simulink model "Basic_cosimulation_circuit_simulator1"  (R2021b)
settings: Solver=ode4  StartTime=0.0  StopTime=inf  FixedStep=Ts  RelTol=1e-3  EnableMultiTasking=on
PostLoadFcn:
  | %
  | % Script for validation of swtiching model design with it's respective
  | % average model.
  | %
  | % Here it is presented the design of the inverter to the 6 kW Fuel Cell
  | % model.
  | 
  | %%% Initialization %%%
  | 
  | 
  | % ------------------------------------- %
  | % ---------- Inverter Design ---------- %
  | % ------------------------------------- %
  | 
  | %%%% Nominal Parameters %%%%
  | 
  | Pnom = 50e3;                                        % Nominal Power
  | Vdc = 400;                                          % DC Voltage - Boost
  | m = 0.6;                                            % Modulation Index
  | Vnom_peak = m*Vdc/2;                                % Peak Voltage
  | Vnom_rms = Vnom_peak/sqrt(2);                       % Rms Voltage
  | FP_min = 0.9;                                       % For Reactive Power
  |                                                     % Compensation
  | Snom = Pnom/FP_min;                                 % Apparent Power
  | Irms = Pnom/(sqrt(3)*Vnom_rms);                     % Rms Curren
  | Inom_peak = Irms*sqrt(2);                           % Peak Current
  | Zbase = Vnom_peak/Inom_peak;                        % Base Impedance
  | f = 60;                                             % Nominal Frequency
  | wnom = 2*pi*60;                                     % Angular Frequency
  | 
  | % ------------------------- %
  | % Inverter LC Filter Design %
  | % ------------------------- %
  | 
  | fsw_inv = 96*60;                                    % Switching Frequency must be a multiple of the nominal frequency
  |                                                      % for proper operation of the Artemis Block
  | ripple_inv = 0.03;
  | L_inv = ((Vdc/2)-Vnom_peak)*(1/fsw_inv)/(ripple_inv*Inom_peak);
  | 
  | % - Capacitor
  | fres = 420;                                         % Filters Ressonant Frequency
  | 
  | Cf = 1/(4*L_inv*(pi^2)*(fres^2));                % Filter Capacitor
  | Rf = 1/(wnom*Cf*50);                                % Damping Resistor
  | 
  | % --- Sample Time --- %
  | 
  | Tsw = 0.00050;
  | Ts = Tsw/10;
  | 
  | % ---------------------- %
  | % Current Control Design %
  | % ---------------------- %
  | 
  | Ron = 0.001;                                        % IGBT Resistance
  | tau_i = 1e-3;                                       % Responde Time
  | kp_current = L_inv/tau_i;                           % PI Proportional Gain
  | ki_current = (Ron)/tau_i;                           % PI Integral Gain
  | 
  | decouple = (wnom*L_inv);                            % Decoupling Gain
InitFcn:
  | %
  | % Script for validation of swtiching model design with it's respective
  | % average model.
  | %
  | % Here it is presented the design of the inverter to the 6 kW Fuel Cell
  | % model.
  | 
  | %%% Initialization %%%
  | 
  | 
  | % ------------------------------------- %
  | % ---------- Inverter Design ---------- %
  | % ------------------------------------- %
  | 
  | %%%% Nominal Parameters %%%%
  | 
  | Pnom = 50e3;                                        % Nominal Power
  | Vdc = 400;                                          % DC Voltage - Boost
  | m = 0.6;                                            % Modulation Index
  | Vnom_peak = m*Vdc/2;                                % Peak Voltage
  | Vnom_rms = Vnom_peak/sqrt(2);                       % Rms Voltage
  | FP_min = 0.9;                                       % For Reactive Power
  |                                                     % Compensation
  | Snom = Pnom/FP_min;                                 % Apparent Power
  | Irms = Pnom/(sqrt(3)*Vnom_rms);                     % Rms Curren
  | Inom_peak = Irms*sqrt(2);                           % Peak Current
  | Zbase = Vnom_peak/Inom_peak;                        % Base Impedance
  | f = 60;                                             % Nominal Frequency
  | wnom = 2*pi*60;                                     % Angular Frequency
  | 
  | % ------------------------- %
  | % Inverter LC Filter Design %
  | % ------------------------- %
  | 
  | fsw_inv = 96*60;                                    % Switching Frequency must be a multiple of the nominal frequency
  |                                                      % for proper operation of the Artemis Block
  | ripple_inv = 0.03;
  | L_inv = ((Vdc/2)-Vnom_peak)*(1/fsw_inv)/(ripple_inv*Inom_peak);
  | 
  | % - Capacitor
  | fres = 420;                                         % Filters Ressonant Frequency
  | 
  | Cf = 1/(4*L_inv*(pi^2)*(fres^2));                % Filter Capacitor
  | Rf = 1/(wnom*Cf*50);                                % Damping Resistor
  | 
  | % --- Sample Time --- %
  | 
  | Tsw = 0.00050;
  | Ts = Tsw/10;
  | 
  | % ---------------------- %
  | % Current Control Design %
  | % ---------------------- %
  | 
  | Ron = 0.001;                                        % IGBT Resistance
  | tau_i = 1e-3;                                       % Responde Time
  | kp_current = L_inv/tau_i;                           % PI Proportional Gain
  | ki_current = (Ron)/tau_i;                           % PI Integral Gain
  | 
  | decouple = (wnom*L_inv);                            % Decoupling Gain
undefined symbols (not defined in the file): D1, Delta, DiscIntNeverNeededParam, IP, j, ph, sps, UDP
libraries: spsCurrentMeasurementLib x25, spsControlledVoltageSourceLib x21, rtlab x18, spsGroundLib x13, spsThreePhaseSeriesRLCBranchLib x13, spsControlledCurrentSourceLib x11, spsVoltageMeasurementLib x10, simulink x8, rteventslib x8, powerlib_meascontrol x7, spsThreePhaseVIMeasurementLib x4, ssn_inverter_model x4
(part 4 of 5)

== system Basic_cosimulation_circuit_simulator1/SM_Master/Circuit_ITM_Source_DP_AW/DP - > EMT/Subsystem2 ==
  In1 : Inport
  Input2 : Inport  Port=2
  Compare To Constant : simulink/Logic and Bit Operations/Compare To Constant  relop=>=  const=2*pi  OutDataTypeStr=boolean
  Constant : Constant  Value=2*pi
  Constant2 : Constant  Value=2*pi*60
  Integrator : Integrator  ExternalReset=rising  InitialConditionSource=external  ShowStatePort=on
  Product4 : Product
  Sin3 : Trigonometry
  Sum : Sum  Inputs=|+-
  Sum4 : Sum  Inputs=|++
  Out1 : Outport
  wires:
  Product4/1 -> Out1/1
  In1/1 -> Product4/1
  Integrator/1 -> Sum4/2
  Input2/1 -> Sum4/1
  Sum4/1 -> Sin3/1
  Sin3/1 -> Product4/2
  Integrator/State -> Sum/1, Compare To Constant/1
  Constant2/1 -> Integrator/1
  Compare To Constant/1 -> Integrator/2
  Sum/1 -> Integrator/3
  Constant/1 -> Sum/2

== system Basic_cosimulation_circuit_simulator1/SM_Master/Original Circuit/Control/Current Control ==
  note: Block Inputs
  Deblock : Inport
  Idq_ref : Inport  Port=2
  Idq : Inport  Port=3
  Vdq : Inport  Port=4
  Phase : Inport  Port=5
  Constant2 : Constant  Value=Vdc/2
  Delay : Delay  DelayLength=1
  Demux1 : Demux  Outputs=2
  Demux2 : Demux  Outputs=2
  Demux3 : Demux  Outputs=2
  Discrete-Time Integrator : DiscreteIntegrator  SampleTime=-1  ICPrevOutput=DiscIntNeverNeededParam  ICPrevScaledInput=DiscIntNeverNeededParam
  Discrete-Time Integrator1 : DiscreteIntegrator  SampleTime=-1  ICPrevOutput=DiscIntNeverNeededParam  ICPrevScaledInput=DiscIntNeverNeededParam
  Divide : Product  Inputs=*/
  Divide1 : Product  Inputs=*/
  Gain1 : Gain  Gain=kp_current
  Gain2 : Gain  Gain=ki_current
  Gain3 : Gain  Gain=kp_current
  Gain4 : Gain  Gain=ki_current
  Gain5 : Gain  Gain=decouple
  Gain6 : Gain  Gain=decouple
  Inverse_Park_Transformation : Subsystem
  Mux : Mux  Inputs=2
  Product : Product
  Product1 : Product
  Saturation : Saturate  UpperLimit=1.2*Inom_peak  LowerLimit=-1.2*Inom_peak
  Saturation1 : Saturate  UpperLimit=1.2*Inom_peak  LowerLimit=-1.2*Inom_peak
  Subtract : Sum  Inputs=+-
  Subtract1 : Sum  Inputs=+-
  Sum1 : Sum
  Sum2 : Sum
  Sum3 : Sum  Inputs=++-
  Sum4 : Sum  Inputs=+++
  modulation : Outport
  wires:
  Sum4/1 -> Divide1/1
  Sum3/1 -> Divide/1
  Sum2/1 -> Sum4/2
  Subtract/1 -> Product/1
  Gain2/1 -> Discrete-Time Integrator/1
  [Iq] -> Gain5/1
  Gain1/1 -> Sum1/1
  [Id] -> Gain6/1
  Subtract1/1 -> Product1/2
  Gain6/1 -> Sum4/1
  Product/1 -> Gain2/1, Gain1/1
  [Vd] -> Sum3/1
  Constant2/1 -> Divide1/2, Divide/2
  Idq_ref/1 -> Demux3/1
  Mux/1 -> Delay/1
  Gain5/1 -> Sum3/3
  Sum1/1 -> Sum3/2
  Discrete-Time Integrator/1 -> Sum1/2
  Gain3/1 -> Sum2/1
  Gain4/1 -> Discrete-Time Integrator1/1
  Discrete-Time Integrator1/1 -> Sum2/2
  [Vq] -> Sum4/3
  Product1/1 -> Gain3/1, Gain4/1
  [Id] -> Subtract/2
  Divide/1 -> Mux/1
  Divide1/1 -> Mux/2
  [Iq] -> Subtract1/2
  Inverse_Park_Transformation/1(ABC) -> modulation/1
  Idq/1 -> Demux1/1
  Demux1/1 -> [Id]
  Demux1/2 -> [Iq]
  Demux2/1 -> [Vd]
  Demux2/2 -> [Vq]
  Vdq/1 -> Demux2/1
  [dblk] -> Product1/1, Product/2
  Deblock/1 -> [dblk]
  Phase/1 -> [phase_pll]
  [phase_pll] -> Inverse_Park_Transformation/2(Phase)
  Demux3/1 -> [Id_ref]
  Demux3/2 -> [Iq_ref]
  [Iq_ref] -> Saturation1/1
  [Id_ref] -> Saturation/1
  Saturation/1 -> Subtract/1
  Saturation1/1 -> Subtract1/1
  Delay/1 -> Inverse_Park_Transformation/1(DQ)

== system Basic_cosimulation_circuit_simulator1/SM_Master/Original Circuit/Control/Meas_3_Wire ==
  AB : Inport
  BC : Inport  Port=2
  Gain10 : Gain  Gain=2
  Gain6 : Gain  Gain=2
  Gain7 : Gain  Gain=1/3
  Gain8 : Gain  Gain=1/3
  Gain9 : Gain  Gain=1/3
  Mux : Mux  Inputs=3
  Sum4 : Sum  Inputs=|++
  Sum5 : Sum  Inputs=-+|
  Sum6 : Sum  Inputs=--|
  ABC : Outport
  wires:
  BC/1 -> Sum4/2, Sum5/2, Gain10/1
  AB/1 -> Gain6/1, Sum5/1, Sum6/2
  Gain7/1 -> Mux/1
  Gain9/1 -> Mux/3
  Sum6/1 -> Gain9/1
  Gain6/1 -> Sum4/1
  Gain8/1 -> Mux/2
  Sum5/1 -> Gain8/1
  Gain10/1 -> Sum6/1
  Sum4/1 -> Gain7/1
  Mux/1 -> ABC/1

== system Basic_cosimulation_circuit_simulator1/SM_Master/Original Circuit/Control/Park_Transformation ==
  note: Park Transformation
  ABC : Inport
  Phase : Inport  Port=2
  Constant{,1..3} (4 alike) : Constant  Value=2*pi/3
  Cos : Trigonometry  Operator=cos
  Cos1 : Trigonometry  Operator=cos
  Cos2 : Trigonometry  Operator=cos
  Cos3 : Trigonometry
  Cos4 : Trigonometry
  Cos5 : Trigonometry
  Delay : Delay  DelayLength=1
  Demux : Demux  Outputs=3
  Gain : Gain  Gain=0.666
  Gain1 : Gain  Gain=-0.666
  Mux : Mux  Inputs=2
  Product{,1..5} (6 alike) : Product
  Sum : Sum  Inputs=|+-
  Sum1 : Sum  Inputs=+++
  Sum2 : Sum  Inputs=|++
  Sum3 : Sum  Inputs=|+-
  Sum4 : Sum  Inputs=+++
  Sum5 : Sum  Inputs=|++
  DQ : Outport
  wires:
  ABC/1 -> Demux/1
  Demux/1 -> [A]
  Demux/2 -> [B]
  Demux/3 -> [C]
  Phase/1 -> [phase]
  [A] -> Product/1
  [phase] -> Cos/1
  Cos/1 -> Product/2
  Product/1 -> Sum1/1
  [B] -> Product1/1
  Product1/1 -> Sum1/2
  [phase] -> Sum/1
  Constant/1 -> Sum/2
  Sum/1 -> Cos1/1
  Cos1/1 -> Product1/2
  Sum2/1 -> Cos2/1
  Constant1/1 -> Sum2/2
  Cos2/1 -> Product2/2
  [phase] -> Sum2/1
  [C] -> Product2/1
  Product2/1 -> Sum1/3
  Sum4/1 -> Gain1/1
  Product5/1 -> Sum4/3
  [C] -> Product5/1
  [phase] -> Sum5/1
  Cos5/1 -> Product5/2
  Constant3/1 -> Sum5/2
  Sum5/1 -> Cos5/1
  Cos4/1 -> Product4/2
  Sum3/1 -> Cos4/1
  Constant2/1 -> Sum3/2
  [phase] -> Sum3/1
  Product4/1 -> Sum4/2
  [B] -> Product4/1
  Product3/1 -> Sum4/1
  Cos3/1 -> Product3/2
  [phase] -> Cos3/1
  [A] -> Product3/1
  Sum1/1 -> Gain/1
  Gain/1 -> [D]
  Gain1/1 -> [Q]
  [D] -> Mux/1
  [Q] -> Mux/2
  Mux/1 -> Delay/1
  Delay/1 -> DQ/1

== system Basic_cosimulation_circuit_simulator1/SM_Master/Original Circuit/Control/Park_Transformation1 ==
  note: Park Transformation
  ABC : Inport
  Phase : Inport  Port=2
  Constant{,1..3} (4 alike) : Constant  Value=2*pi/3
  Cos : Trigonometry  Operator=cos
  Cos1 : Trigonometry  Operator=cos
  Cos2 : Trigonometry  Operator=cos
  Cos3 : Trigonometry
  Cos4 : Trigonometry
  Cos5 : Trigonometry
  Delay : Delay  DelayLength=1
  Demux : Demux  Outputs=3
  Gain : Gain  Gain=0.666
  Gain1 : Gain  Gain=-0.666
  Mux : Mux  Inputs=2
  Product{,1..5} (6 alike) : Product
  Sum : Sum  Inputs=|+-
  Sum1 : Sum  Inputs=+++
  Sum2 : Sum  Inputs=|++
  Sum3 : Sum  Inputs=|+-
  Sum4 : Sum  Inputs=+++
  Sum5 : Sum  Inputs=|++
  DQ : Outport
  wires:
  [Q] -> Mux/2
  [D] -> Mux/1
  Gain1/1 -> [Q]
  Gain/1 -> [D]
  Sum1/1 -> Gain/1
  [A] -> Product3/1
  [phase] -> Cos3/1
  Cos3/1 -> Product3/2
  Product3/1 -> Sum4/1
  [B] -> Product4/1
  Product4/1 -> Sum4/2
  [phase] -> Sum3/1
  Constant2/1 -> Sum3/2
  Sum3/1 -> Cos4/1
  Cos4/1 -> Product4/2
  Sum5/1 -> Cos5/1
  Constant3/1 -> Sum5/2
  Cos5/1 -> Product5/2
  [phase] -> Sum5/1
  [C] -> Product5/1
  Product5/1 -> Sum4/3
  Sum4/1 -> Gain1/1
  Product2/1 -> Sum1/3
  [C] -> Product2/1
  [phase] -> Sum2/1
  Cos2/1 -> Product2/2
  Constant1/1 -> Sum2/2
  Sum2/1 -> Cos2/1
  Cos1/1 -> Product1/2
  Sum/1 -> Cos1/1
  Constant/1 -> Sum/2
  [phase] -> Sum/1
  Product1/1 -> Sum1/2
  [B] -> Product1/1
  Product/1 -> Sum1/1
  Cos/1 -> Product/2
  [phase] -> Cos/1
  [A] -> Product/1
  Phase/1 -> [phase]
  Demux/3 -> [C]
  Demux/2 -> [B]
  Demux/1 -> [A]
  ABC/1 -> Demux/1
  Mux/1 -> Delay/1
  Delay/1 -> DQ/1

== system Basic_cosimulation_circuit_simulator1/SM_Master/Original Circuit/Control/Power Control ==
  PQ_ref : Inport
  Vd : Inport  Port=2
  Dblk : Inport  Port=3
  Constant : Constant  Value=Vnom_peak
  Demux2 : Demux  Outputs=2
  Divide : Product  Inputs=*/
  Divide1 : Product  Inputs=*/
  Gain : Gain  Gain=3
  Gain1 : Gain  Gain=2
  Gain2 : Gain  Gain=3
  Gain3 : Gain  Gain=-2
  Mux : Mux  Inputs=2
  Scope : Scope
  Switch : Switch  Criteria=u2 > Threshold
  Transfer Fcn : TransferFcn  Commented=on  Denominator=[0.01 1]
  Out1 : Outport
  wires:
  Gain/1 -> Divide/2
  Demux2/2 -> Gain3/1
  Gain2/1 -> Divide1/2
  Gain3/1 -> Divide1/1
  Demux2/1 -> Gain1/1
  Dblk/1 -> Switch/2
  Gain1/1 -> Divide/1
  Divide/1 -> Mux/1
  Constant/1 -> Switch/3
  [Vd_power] -> Gain/1
  Divide1/1 -> Mux/2
  Mux/1 -> Out1/1
  PQ_ref/1 -> Demux2/1
  Vd/1 -> Switch/1
  Switch/1 -> Scope/1, Gain2/1, [Vd_power]

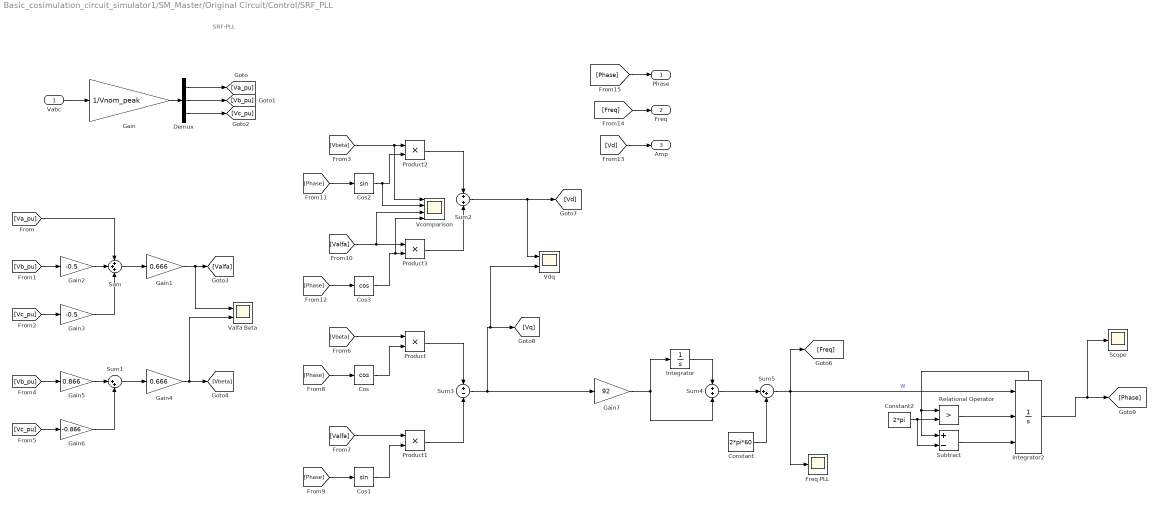
== system Basic_cosimulation_circuit_simulator1/SM_Master/Original Circuit/Control/SRF_PLL ==
  note: SRF-PLL
  Vabc : Inport
  Constant : Constant  Value=2*pi*60
  Constant2 : Constant  Value=2*pi
  Cos : Trigonometry  Operator=cos
  Cos1 : Trigonometry
  Cos2 : Trigonometry
  Cos3 : Trigonometry  Operator=cos
  Demux : Demux  Outputs=3
  Freq PLL : Scope
  Gain : Gain  Gain=1/Vnom_peak
  Gain1 : Gain  Gain=0.666
  Gain2 : Gain  Gain=-0.5
  Gain3 : Gain  Gain=-0.5
  Gain4 : Gain  Gain=0.666
  Gain5 : Gain  Gain=0.866
  Gain6 : Gain  Gain=-0.866
  Gain7 : Gain  Gain=92
  Integrator : Integrator
  Integrator2 : Integrator  ExternalReset=rising  InitialConditionSource=external  InitialCondition=sps.Phase_Init*pi/180  LimitOutput=on  ShowStatePort=on
  Product{,1..3} (4 alike) : Product
  Relational Operator : RelationalOperator  Operator=>  OutDataTypeStr=boolean  RndMeth=Nearest
  Scope : Scope
  Subtract : Sum  Inputs=+-
  Sum : Sum  Inputs=+++
  Sum1 : Sum  Inputs=|++
  Sum2 : Sum  Inputs=+|+
  Sum3 : Sum  Inputs=+|-
  Sum4 : Sum  Inputs=+|+
  Sum5 : Sum  Inputs=|++
  Valfa Beta : Scope  NumInputPorts=2
  Vcomparison : Scope  NumInputPorts=4
  Vdq : Scope  NumInputPorts=2
  Phase : Outport
  Freq : Outport  Port=2
  Amp : Outport  Port=3
  wires:
  Vabc/1 -> Gain/1
  Demux/1 -> [Va_pu]
  Demux/2 -> [Vb_pu]
  Demux/3 -> [Vc_pu]
  Gain/1 -> Demux/1
  Sum/1 -> Gain1/1
  [Va_pu] -> Sum/1
  [Vb_pu] -> Gain2/1
  Gain2/1 -> Sum/2
  [Vc_pu] -> Gain3/1
  Gain3/1 -> Sum/3
  [Vc_pu] -> Gain6/1
  [Vb_pu] -> Gain5/1
  Sum1/1 -> Gain4/1
  Gain4/1 -> Valfa Beta/2, [Vbeta]
  Gain5/1 -> Sum1/1
  Gain6/1 -> Sum1/2
  [Vbeta] -> Product/1
  Product/1 -> Sum3/1
  [Valfa] -> Product1/1
  Product1/1 -> Sum3/2
  Sum3/1 -> Gain7/1, Vdq/2, [Vq]
  Gain7/1 -> Sum4/2, Integrator/1
  Integrator/1 -> Sum4/1
  Sum4/1 -> Sum5/1
  Constant/1 -> Sum5/2
  [Phase] -> Cos/1
  Cos/1 -> Product/2
  [Phase] -> Cos1/1
  Cos1/1 -> Product1/2
  Cos3/1 -> Vcomparison/4, Product3/2
  [Phase] -> Cos3/1
  Cos2/1 -> Vcomparison/2, Product2/2
  [Phase] -> Cos2/1
  Product3/1 -> Sum2/2
  [Valfa] -> Vcomparison/3, Product3/1
  Product2/1 -> Sum2/1
  [Vbeta] -> Vcomparison/1, Product2/1
  [Vd] -> Amp/1
  [Freq] -> Freq/1
  [Phase] -> Phase/1
  Gain1/1 -> Valfa Beta/1, [Valfa]
  Sum2/1 -> Vdq/1, [Vd]
  Integrator2/1 -> Scope/1, [Phase]
  Subtract/1 -> Integrator2/3
  Integrator2/State -> Relational Operator/1, Subtract/1
  Sum5/1 -> Integrator2/1, Freq PLL/1, [Freq]  "W"
  Relational Operator/1 -> Integrator2/2
  Constant2/1 -> Relational Operator/2, Subtract/2

== system Basic_cosimulation_circuit_simulator1/SM_Master/VSC_ITM_Average_Moving_Window/Control/Current Control ==
  note: Block Inputs
  Deblock : Inport
  Idq_ref : Inport  Port=2
  Idq : Inport  Port=3
  Vdq : Inport  Port=4
  Phase : Inport  Port=5
  Constant2 : Constant  Value=Vdc/2
  Delay : Delay  DelayLength=1
  Demux1 : Demux  Outputs=2
  Demux2 : Demux  Outputs=2
  Demux3 : Demux  Outputs=2
  Discrete-Time Integrator : DiscreteIntegrator  SampleTime=-1  ICPrevOutput=DiscIntNeverNeededParam  ICPrevScaledInput=DiscIntNeverNeededParam
  Discrete-Time Integrator1 : DiscreteIntegrator  SampleTime=-1  ICPrevOutput=DiscIntNeverNeededParam  ICPrevScaledInput=DiscIntNeverNeededParam
  Divide : Product  Inputs=*/
  Divide1 : Product  Inputs=*/
  Gain1 : Gain  Gain=kp_current
  Gain2 : Gain  Gain=ki_current
  Gain3 : Gain  Gain=kp_current
  Gain4 : Gain  Gain=ki_current
  Gain5 : Gain  Gain=decouple
  Gain6 : Gain  Gain=decouple
  Inverse_Park_Transformation : Subsystem
  Mux : Mux  Inputs=2
  Product : Product
  Product1 : Product
  Saturation : Saturate  UpperLimit=1.2*Inom_peak  LowerLimit=-1.2*Inom_peak
  Saturation1 : Saturate  UpperLimit=1.2*Inom_peak  LowerLimit=-1.2*Inom_peak
  Scope : Scope  Commented=on
  Subtract : Sum  Inputs=+-
  Subtract1 : Sum  Inputs=+-
  Sum1 : Sum
  Sum2 : Sum
  Sum3 : Sum  Inputs=++-
  Sum4 : Sum  Inputs=+++
  modulation : Outport
  wires:
  Sum4/1 -> Divide1/1
  Sum3/1 -> Divide/1
  Sum2/1 -> Sum4/2
  Subtract/1 -> Product/1
  Gain2/1 -> Discrete-Time Integrator/1
  [Iq] -> Gain5/1
  Gain1/1 -> Sum1/1
  [Id] -> Gain6/1
  Subtract1/1 -> Product1/2
  Gain6/1 -> Sum4/1
  Product/1 -> Gain2/1, Gain1/1
  [Vd] -> Sum3/1
  Constant2/1 -> Divide1/2, Divide/2
  Idq_ref/1 -> Demux3/1
  Mux/1 -> Delay/1
  Gain5/1 -> Sum3/3
  Sum1/1 -> Sum3/2
  Discrete-Time Integrator/1 -> Sum1/2
  Gain3/1 -> Sum2/1
  Gain4/1 -> Discrete-Time Integrator1/1
  Discrete-Time Integrator1/1 -> Sum2/2
  [Vq] -> Sum4/3
  Product1/1 -> Gain3/1, Gain4/1
  [Id] -> Subtract/2
  Divide/1 -> Mux/1
  Divide1/1 -> Mux/2
  [Iq] -> Subtract1/2
  Inverse_Park_Transformation/1(ABC) -> modulation/1
  Idq/1 -> Demux1/1
  Demux1/1 -> [Id]
  Demux1/2 -> [Iq]
  Demux2/1 -> [Vd]
  Demux2/2 -> [Vq]
  Vdq/1 -> Demux2/1
  [dblk] -> Product1/1, Product/2
  Deblock/1 -> [dblk]
  Phase/1 -> [phase_pll]
  [phase_pll] -> Inverse_Park_Transformation/2(Phase)
  Demux3/1 -> [Id_ref]
  Demux3/2 -> [Iq_ref]
  [Iq_ref] -> Saturation1/1
  [Id_ref] -> Saturation/1
  Saturation/1 -> Subtract/1
  Saturation1/1 -> Subtract1/1
  Delay/1 -> Scope/1, Inverse_Park_Transformation/1(DQ)

== system Basic_cosimulation_circuit_simulator1/SM_Master/VSC_ITM_Average_Moving_Window/Control/Meas_3_Wire ==
  AB : Inport
  BC : Inport  Port=2
  Gain10 : Gain  Gain=2
  Gain6 : Gain  Gain=2
  Gain7 : Gain  Gain=1/3
  Gain8 : Gain  Gain=1/3
  Gain9 : Gain  Gain=1/3
  Mux : Mux  Inputs=3
  Sum4 : Sum  Inputs=|++
  Sum5 : Sum  Inputs=-+|
  Sum6 : Sum  Inputs=--|
  ABC : Outport
  wires:
  BC/1 -> Sum4/2, Sum5/2, Gain10/1
  AB/1 -> Gain6/1, Sum5/1, Sum6/2
  Gain7/1 -> Mux/1
  Gain9/1 -> Mux/3
  Sum6/1 -> Gain9/1
  Gain6/1 -> Sum4/1
  Gain8/1 -> Mux/2
  Sum5/1 -> Gain8/1
  Gain10/1 -> Sum6/1
  Sum4/1 -> Gain7/1
  Mux/1 -> ABC/1

== system Basic_cosimulation_circuit_simulator1/SM_Master/VSC_ITM_Average_Moving_Window/Control/Park_Transformation ==
  note: Park Transformation
  ABC : Inport
  Phase : Inport  Port=2
  Constant{,1..3} (4 alike) : Constant  Value=2*pi/3
  Cos : Trigonometry  Operator=cos
  Cos1 : Trigonometry  Operator=cos
  Cos2 : Trigonometry  Operator=cos
  Cos3 : Trigonometry
  Cos4 : Trigonometry
  Cos5 : Trigonometry
  Delay : Delay  DelayLength=1
  Demux : Demux  Outputs=3
  Gain : Gain  Gain=0.666
  Gain1 : Gain  Gain=-0.666
  Mux : Mux  Inputs=2
  Product{,1..5} (6 alike) : Product
  Sum : Sum  Inputs=|+-
  Sum1 : Sum  Inputs=+++
  Sum2 : Sum  Inputs=|++
  Sum3 : Sum  Inputs=|+-
  Sum4 : Sum  Inputs=+++
  Sum5 : Sum  Inputs=|++
  DQ : Outport
  wires:
  ABC/1 -> Demux/1
  Demux/1 -> [A]
  Demux/2 -> [B]
  Demux/3 -> [C]
  Phase/1 -> [phase]
  [A] -> Product/1
  [phase] -> Cos/1
  Cos/1 -> Product/2
  Product/1 -> Sum1/1
  [B] -> Product1/1
  Product1/1 -> Sum1/2
  [phase] -> Sum/1
  Constant/1 -> Sum/2
  Sum/1 -> Cos1/1
  Cos1/1 -> Product1/2
  Sum2/1 -> Cos2/1
  Constant1/1 -> Sum2/2
  Cos2/1 -> Product2/2
  [phase] -> Sum2/1
  [C] -> Product2/1
  Product2/1 -> Sum1/3
  Sum4/1 -> Gain1/1
  Product5/1 -> Sum4/3
  [C] -> Product5/1
  [phase] -> Sum5/1
  Cos5/1 -> Product5/2
  Constant3/1 -> Sum5/2
  Sum5/1 -> Cos5/1
  Cos4/1 -> Product4/2
  Sum3/1 -> Cos4/1
  Constant2/1 -> Sum3/2
  [phase] -> Sum3/1
  Product4/1 -> Sum4/2
  [B] -> Product4/1
  Product3/1 -> Sum4/1
  Cos3/1 -> Product3/2
  [phase] -> Cos3/1
  [A] -> Product3/1
  Sum1/1 -> Gain/1
  Gain/1 -> [D]
  Gain1/1 -> [Q]
  [D] -> Mux/1
  [Q] -> Mux/2
  Mux/1 -> Delay/1
  Delay/1 -> DQ/1

== system Basic_cosimulation_circuit_simulator1/SM_Master/VSC_ITM_Average_Moving_Window/Control/Park_Transformation1 ==
  note: Park Transformation
  ABC : Inport
  Phase : Inport  Port=2
  Constant{,1..3} (4 alike) : Constant  Value=2*pi/3
  Cos : Trigonometry  Operator=cos
  Cos1 : Trigonometry  Operator=cos
  Cos2 : Trigonometry  Operator=cos
  Cos3 : Trigonometry
  Cos4 : Trigonometry
  Cos5 : Trigonometry
  Delay : Delay  DelayLength=1
  Demux : Demux  Outputs=3
  Gain : Gain  Gain=0.666
  Gain1 : Gain  Gain=-0.666
  Mux : Mux  Inputs=2
  Product{,1..5} (6 alike) : Product
  Sum : Sum  Inputs=|+-
  Sum1 : Sum  Inputs=+++
  Sum2 : Sum  Inputs=|++
  Sum3 : Sum  Inputs=|+-
  Sum4 : Sum  Inputs=+++
  Sum5 : Sum  Inputs=|++
  DQ : Outport
  wires:
  [Q] -> Mux/2
  [D] -> Mux/1
  Gain1/1 -> [Q]
  Gain/1 -> [D]
  Sum1/1 -> Gain/1
  [A] -> Product3/1
  [phase] -> Cos3/1
  Cos3/1 -> Product3/2
  Product3/1 -> Sum4/1
  [B] -> Product4/1
  Product4/1 -> Sum4/2
  [phase] -> Sum3/1
  Constant2/1 -> Sum3/2
  Sum3/1 -> Cos4/1
  Cos4/1 -> Product4/2
  Sum5/1 -> Cos5/1
  Constant3/1 -> Sum5/2
  Cos5/1 -> Product5/2
  [phase] -> Sum5/1
  [C] -> Product5/1
  Product5/1 -> Sum4/3
  Sum4/1 -> Gain1/1
  Product2/1 -> Sum1/3
  [C] -> Product2/1
  [phase] -> Sum2/1
  Cos2/1 -> Product2/2
  Constant1/1 -> Sum2/2
  Sum2/1 -> Cos2/1
  Cos1/1 -> Product1/2
  Sum/1 -> Cos1/1
  Constant/1 -> Sum/2
  [phase] -> Sum/1
  Product1/1 -> Sum1/2
  [B] -> Product1/1
  Product/1 -> Sum1/1
  Cos/1 -> Product/2
  [phase] -> Cos/1
  [A] -> Product/1
  Phase/1 -> [phase]
  Demux/3 -> [C]
  Demux/2 -> [B]
  Demux/1 -> [A]
  ABC/1 -> Demux/1
  Mux/1 -> Delay/1
  Delay/1 -> DQ/1

== system Basic_cosimulation_circuit_simulator1/SM_Master/VSC_ITM_Average_Moving_Window/Control/Power Control ==
  PQ_ref : Inport
  Vd : Inport  Port=2
  Dblk : Inport  Port=3
  Constant : Constant  Value=Vnom_peak
  Demux2 : Demux  Outputs=2
  Divide : Product  Inputs=*/
  Divide1 : Product  Inputs=*/
  Gain : Gain  Gain=3
  Gain1 : Gain  Gain=2
  Gain2 : Gain  Gain=3
  Gain3 : Gain  Gain=-2
  Mux : Mux  Inputs=2
  Scope : Scope
  Switch : Switch  Criteria=u2 > Threshold
  Transfer Fcn : TransferFcn  Commented=on  Denominator=[0.01 1]
  Out1 : Outport
  wires:
  Gain/1 -> Divide/2
  Demux2/2 -> Gain3/1
  Gain2/1 -> Divide1/2
  Gain3/1 -> Divide1/1
  Demux2/1 -> Gain1/1
  Dblk/1 -> Switch/2
  Gain1/1 -> Divide/1
  Divide/1 -> Mux/1
  Constant/1 -> Switch/3
  [Vd_power] -> Gain/1
  Divide1/1 -> Mux/2
  Mux/1 -> Out1/1
  PQ_ref/1 -> Demux2/1
  Vd/1 -> Switch/1
  Switch/1 -> Scope/1, Gain2/1, [Vd_power]

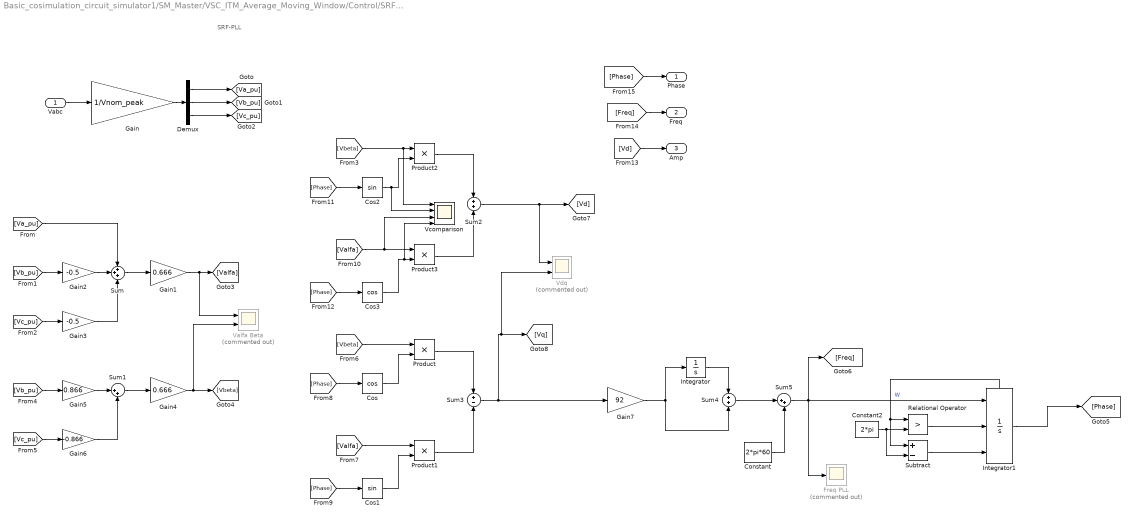
== system Basic_cosimulation_circuit_simulator1/SM_Master/VSC_ITM_Average_Moving_Window/Control/SRF_PLL ==
  note: SRF-PLL
  Vabc : Inport
  Constant : Constant  Value=2*pi*60
  Constant2 : Constant  Value=2*pi
  Cos : Trigonometry  Operator=cos
  Cos1 : Trigonometry
  Cos2 : Trigonometry
  Cos3 : Trigonometry  Operator=cos
  Demux : Demux  Outputs=3
  Freq PLL : Scope  Commented=on
  Gain : Gain  Gain=1/Vnom_peak
  Gain1 : Gain  Gain=0.666
  Gain2 : Gain  Gain=-0.5
  Gain3 : Gain  Gain=-0.5
  Gain4 : Gain  Gain=0.666
  Gain5 : Gain  Gain=0.866
  Gain6 : Gain  Gain=-0.866
  Gain7 : Gain  Gain=92
  Integrator : Integrator
  Integrator1 : Integrator  ExternalReset=rising  InitialConditionSource=external  InitialCondition=sps.Phase_Init*pi/180  LimitOutput=on  ShowStatePort=on
  Product{,1..3} (4 alike) : Product
  Relational Operator : RelationalOperator  Operator=>  OutDataTypeStr=boolean  RndMeth=Nearest
  Subtract : Sum  Inputs=+-
  Sum : Sum  Inputs=+++
  Sum1 : Sum  Inputs=|++
  Sum2 : Sum  Inputs=+|+
  Sum3 : Sum  Inputs=+|-
  Sum4 : Sum  Inputs=+|+
  Sum5 : Sum  Inputs=|++
  Valfa Beta : Scope  Commented=on  NumInputPorts=2
  Vcomparison : Scope  NumInputPorts=4
  Vdq : Scope  Commented=on  NumInputPorts=2
  Phase : Outport
  Freq : Outport  Port=2
  Amp : Outport  Port=3
  wires:
  Vabc/1 -> Gain/1
  Demux/1 -> [Va_pu]
  Demux/2 -> [Vb_pu]
  Demux/3 -> [Vc_pu]
  Gain/1 -> Demux/1
  Sum/1 -> Gain1/1
  [Va_pu] -> Sum/1
  [Vb_pu] -> Gain2/1
  Gain2/1 -> Sum/2
  [Vc_pu] -> Gain3/1
  Gain3/1 -> Sum/3
  [Vc_pu] -> Gain6/1
  [Vb_pu] -> Gain5/1
  Sum1/1 -> Gain4/1
  Gain4/1 -> Valfa Beta/2, [Vbeta]
  Gain5/1 -> Sum1/1
  Gain6/1 -> Sum1/2
  [Vbeta] -> Product/1
  Product/1 -> Sum3/1
  [Valfa] -> Product1/1
  Product1/1 -> Sum3/2
  Sum3/1 -> Gain7/1, Vdq/2, [Vq]
  Gain7/1 -> Sum4/2, Integrator/1
  Integrator/1 -> Sum4/1
  Sum4/1 -> Sum5/1
  Constant/1 -> Sum5/2
  [Phase] -> Cos/1
  Cos/1 -> Product/2
  [Phase] -> Cos1/1
  Cos1/1 -> Product1/2
  Cos3/1 -> Vcomparison/4, Product3/2
  [Phase] -> Cos3/1
  Cos2/1 -> Vcomparison/2, Product2/2
  [Phase] -> Cos2/1
  Product3/1 -> Sum2/2
  [Valfa] -> Vcomparison/3, Product3/1
  Product2/1 -> Sum2/1
  [Vbeta] -> Vcomparison/1, Product2/1
  [Vd] -> Amp/1
  [Freq] -> Freq/1
  [Phase] -> Phase/1
  Gain1/1 -> Valfa Beta/1, [Valfa]
  Sum2/1 -> Vdq/1, [Vd]
  Constant2/1 -> Relational Operator/2, Subtract/2
  Integrator1/State -> Relational Operator/1, Subtract/1
  Sum5/1 -> Integrator1/1, Freq PLL/1, [Freq]  "W"
  Relational Operator/1 -> Integrator1/2
  Subtract/1 -> Integrator1/3
  Integrator1/1 -> [Phase]

== system Basic_cosimulation_circuit_simulator1/SM_Master/VSC_ITM_Average_Moving_Window/DP - > EMT/Subsystem ==
  In1 : Inport
  Input : Inport  Port=2
  Compare To Constant : simulink/Logic and Bit Operations/Compare To Constant  relop=>=  const=2*pi  OutDataTypeStr=boolean
  Constant : Constant  Value=2*pi
  Constant2 : Constant  Value=2*pi*60
  Integrator : Integrator  ExternalReset=rising  InitialConditionSource=external  ShowStatePort=on
  Product4 : Product
  Sin3 : Trigonometry
  Sum : Sum  Inputs=|+-
  Sum4 : Sum  Inputs=|++
  Out1 : Outport
  wires:
  Product4/1 -> Out1/1
  In1/1 -> Product4/1
  Integrator/1 -> Sum4/2
  Input/1 -> Sum4/1
  Sum4/1 -> Sin3/1
  Sin3/1 -> Product4/2
  Integrator/State -> Sum/1, Compare To Constant/1
  Constant2/1 -> Integrator/1
  Compare To Constant/1 -> Integrator/2
  Sum/1 -> Integrator/3
  Constant/1 -> Sum/2

== system Basic_cosimulation_circuit_simulator1/SM_Master/VSC_ITM_Average_Moving_Window/DP - > EMT/Subsystem1 ==
  In1 : Inport
  Input1 : Inport  Port=2
  Compare To Constant : simulink/Logic and Bit Operations/Compare To Constant  relop=>=  const=2*pi  OutDataTypeStr=boolean
  Constant : Constant  Value=2*pi
  Constant2 : Constant  Value=2*pi*60
  Integrator : Integrator  ExternalReset=rising  InitialConditionSource=external  ShowStatePort=on
  Product4 : Product
  Sin3 : Trigonometry
  Sum : Sum  Inputs=|+-
  Sum4 : Sum  Inputs=|++
  Out1 : Outport
  wires:
  Product4/1 -> Out1/1
  In1/1 -> Product4/1
  Integrator/1 -> Sum4/2
  Input1/1 -> Sum4/1
  Sum4/1 -> Sin3/1
  Sin3/1 -> Product4/2
  Constant/1 -> Sum/2
  Sum/1 -> Integrator/3
  Compare To Constant/1 -> Integrator/2
  Integrator/State -> Sum/1, Compare To Constant/1
  Constant2/1 -> Integrator/1

== system Basic_cosimulation_circuit_simulator1/SM_Master/VSC_ITM_Average_Moving_Window/DP - > EMT/Subsystem2 ==
  In1 : Inport
  Input2 : Inport  Port=2
  Compare To Constant : simulink/Logic and Bit Operations/Compare To Constant  relop=>=  const=2*pi  OutDataTypeStr=boolean
  Constant : Constant  Value=2*pi
  Constant2 : Constant  Value=2*pi*60
  Integrator : Integrator  ExternalReset=rising  InitialConditionSource=external  ShowStatePort=on
  Product4 : Product
  Sin3 : Trigonometry
  Sum : Sum  Inputs=|+-
  Sum4 : Sum  Inputs=|++
  Out1 : Outport
  wires:
  Product4/1 -> Out1/1
  In1/1 -> Product4/1
  Integrator/1 -> Sum4/2
  Input2/1 -> Sum4/1
  Sum4/1 -> Sin3/1
  Sin3/1 -> Product4/2
  Integrator/State -> Sum/1, Compare To Constant/1
  Constant2/1 -> Integrator/1
  Compare To Constant/1 -> Integrator/2
  Sum/1 -> Integrator/3
  Constant/1 -> Sum/2

== system Basic_cosimulation_circuit_simulator1/SM_Master/VSC_ITM_Intantaneous_values/Control/Current Control ==
  note: Block Inputs
  Deblock : Inport
  Idq_ref : Inport  Port=2
  Idq : Inport  Port=3
  Vdq : Inport  Port=4
  Phase : Inport  Port=5
  Constant2 : Constant  Value=Vdc/2
  Delay : Delay  DelayLength=1
  Demux1 : Demux  Outputs=2
  Demux2 : Demux  Outputs=2
  Demux3 : Demux  Outputs=2
  Discrete-Time Integrator : DiscreteIntegrator  SampleTime=-1  ICPrevOutput=DiscIntNeverNeededParam  ICPrevScaledInput=DiscIntNeverNeededParam
  Discrete-Time Integrator1 : DiscreteIntegrator  SampleTime=-1  ICPrevOutput=DiscIntNeverNeededParam  ICPrevScaledInput=DiscIntNeverNeededParam
  Divide : Product  Inputs=*/
  Divide1 : Product  Inputs=*/
  Gain1 : Gain  Gain=kp_current
  Gain2 : Gain  Gain=ki_current
  Gain3 : Gain  Gain=kp_current
  Gain4 : Gain  Gain=ki_current
  Gain5 : Gain  Gain=decouple
  Gain6 : Gain  Gain=decouple
  Inverse_Park_Transformation : Subsystem
  Mux : Mux  Inputs=2
  Product : Product
  Product1 : Product
  Saturation : Saturate  UpperLimit=1.2*Inom_peak  LowerLimit=-1.2*Inom_peak
  Saturation1 : Saturate  UpperLimit=1.2*Inom_peak  LowerLimit=-1.2*Inom_peak
  Scope : Scope  Commented=on
  Subtract : Sum  Inputs=+-
  Subtract1 : Sum  Inputs=+-
  Sum1 : Sum
  Sum2 : Sum
  Sum3 : Sum  Inputs=++-
  Sum4 : Sum  Inputs=+++
  modulation : Outport
  wires:
  Sum4/1 -> Divide1/1
  Sum3/1 -> Divide/1
  Sum2/1 -> Sum4/2
  Subtract/1 -> Product/1
  Gain2/1 -> Discrete-Time Integrator/1
  [Iq] -> Gain5/1
  Gain1/1 -> Sum1/1
  [Id] -> Gain6/1
  Subtract1/1 -> Product1/2
  Gain6/1 -> Sum4/1
  Product/1 -> Gain2/1, Gain1/1
  [Vd] -> Sum3/1
  Constant2/1 -> Divide1/2, Divide/2
  Idq_ref/1 -> Demux3/1
  Mux/1 -> Delay/1
  Gain5/1 -> Sum3/3
  Sum1/1 -> Sum3/2
  Discrete-Time Integrator/1 -> Sum1/2
  Gain3/1 -> Sum2/1
  Gain4/1 -> Discrete-Time Integrator1/1
  Discrete-Time Integrator1/1 -> Sum2/2
  [Vq] -> Sum4/3
  Product1/1 -> Gain3/1, Gain4/1
  [Id] -> Subtract/2
  Divide/1 -> Mux/1
  Divide1/1 -> Mux/2
  [Iq] -> Subtract1/2
  Inverse_Park_Transformation/1(ABC) -> modulation/1
  Idq/1 -> Demux1/1
  Demux1/1 -> [Id]
  Demux1/2 -> [Iq]
  Demux2/1 -> [Vd]
  Demux2/2 -> [Vq]
  Vdq/1 -> Demux2/1
  [dblk] -> Product1/1, Product/2
  Deblock/1 -> [dblk]
  Phase/1 -> [phase_pll]
  [phase_pll] -> Inverse_Park_Transformation/2(Phase)
  Demux3/1 -> [Id_ref]
  Demux3/2 -> [Iq_ref]
  [Iq_ref] -> Saturation1/1
  [Id_ref] -> Saturation/1
  Saturation/1 -> Subtract/1
  Saturation1/1 -> Subtract1/1
  Delay/1 -> Scope/1, Inverse_Park_Transformation/1(DQ)

== system Basic_cosimulation_circuit_simulator1/SM_Master/VSC_ITM_Intantaneous_values/Control/Meas_3_Wire ==
  AB : Inport
  BC : Inport  Port=2
  Gain10 : Gain  Gain=2
  Gain6 : Gain  Gain=2
  Gain7 : Gain  Gain=1/3
  Gain8 : Gain  Gain=1/3
  Gain9 : Gain  Gain=1/3
  Mux : Mux  Inputs=3
  Sum4 : Sum  Inputs=|++
  Sum5 : Sum  Inputs=-+|
  Sum6 : Sum  Inputs=--|
  ABC : Outport
  wires:
  BC/1 -> Sum4/2, Sum5/2, Gain10/1
  AB/1 -> Gain6/1, Sum5/1, Sum6/2
  Gain7/1 -> Mux/1
  Gain9/1 -> Mux/3
  Sum6/1 -> Gain9/1
  Gain6/1 -> Sum4/1
  Gain8/1 -> Mux/2
  Sum5/1 -> Gain8/1
  Gain10/1 -> Sum6/1
  Sum4/1 -> Gain7/1
  Mux/1 -> ABC/1

== system Basic_cosimulation_circuit_simulator1/SM_Master/VSC_ITM_Intantaneous_values/Control/Park_Transformation ==
  note: Park Transformation
  ABC : Inport
  Phase : Inport  Port=2
  Constant{,1..3} (4 alike) : Constant  Value=2*pi/3
  Cos : Trigonometry  Operator=cos
  Cos1 : Trigonometry  Operator=cos
  Cos2 : Trigonometry  Operator=cos
  Cos3 : Trigonometry
  Cos4 : Trigonometry
  Cos5 : Trigonometry
  Delay : Delay  DelayLength=1
  Demux : Demux  Outputs=3
  Gain : Gain  Gain=0.666
  Gain1 : Gain  Gain=-0.666
  Mux : Mux  Inputs=2
  Product{,1..5} (6 alike) : Product
  Sum : Sum  Inputs=|+-
  Sum1 : Sum  Inputs=+++
  Sum2 : Sum  Inputs=|++
  Sum3 : Sum  Inputs=|+-
  Sum4 : Sum  Inputs=+++
  Sum5 : Sum  Inputs=|++
  DQ : Outport
  wires:
  ABC/1 -> Demux/1
  Demux/1 -> [A]
  Demux/2 -> [B]
  Demux/3 -> [C]
  Phase/1 -> [phase]
  [A] -> Product/1
  [phase] -> Cos/1
  Cos/1 -> Product/2
  Product/1 -> Sum1/1
  [B] -> Product1/1
  Product1/1 -> Sum1/2
  [phase] -> Sum/1
  Constant/1 -> Sum/2
  Sum/1 -> Cos1/1
  Cos1/1 -> Product1/2
  Sum2/1 -> Cos2/1
  Constant1/1 -> Sum2/2
  Cos2/1 -> Product2/2
  [phase] -> Sum2/1
  [C] -> Product2/1
  Product2/1 -> Sum1/3
  Sum4/1 -> Gain1/1
  Product5/1 -> Sum4/3
  [C] -> Product5/1
  [phase] -> Sum5/1
  Cos5/1 -> Product5/2
  Constant3/1 -> Sum5/2
  Sum5/1 -> Cos5/1
  Cos4/1 -> Product4/2
  Sum3/1 -> Cos4/1
  Constant2/1 -> Sum3/2
  [phase] -> Sum3/1
  Product4/1 -> Sum4/2
  [B] -> Product4/1
  Product3/1 -> Sum4/1
  Cos3/1 -> Product3/2
  [phase] -> Cos3/1
  [A] -> Product3/1
  Sum1/1 -> Gain/1
  Gain/1 -> [D]
  Gain1/1 -> [Q]
  [D] -> Mux/1
  [Q] -> Mux/2
  Mux/1 -> Delay/1
  Delay/1 -> DQ/1

== system Basic_cosimulation_circuit_simulator1/SM_Master/VSC_ITM_Intantaneous_values/Control/Park_Transformation1 ==
  note: Park Transformation
  ABC : Inport
  Phase : Inport  Port=2
  Constant{,1..3} (4 alike) : Constant  Value=2*pi/3
  Cos : Trigonometry  Operator=cos
  Cos1 : Trigonometry  Operator=cos
  Cos2 : Trigonometry  Operator=cos
  Cos3 : Trigonometry
  Cos4 : Trigonometry
  Cos5 : Trigonometry
  Delay : Delay  DelayLength=1
  Demux : Demux  Outputs=3
  Gain : Gain  Gain=0.666
  Gain1 : Gain  Gain=-0.666
  Mux : Mux  Inputs=2
  Product{,1..5} (6 alike) : Product
  Sum : Sum  Inputs=|+-
  Sum1 : Sum  Inputs=+++
  Sum2 : Sum  Inputs=|++
  Sum3 : Sum  Inputs=|+-
  Sum4 : Sum  Inputs=+++
  Sum5 : Sum  Inputs=|++
  DQ : Outport
  wires:
  [Q] -> Mux/2
  [D] -> Mux/1
  Gain1/1 -> [Q]
  Gain/1 -> [D]
  Sum1/1 -> Gain/1
  [A] -> Product3/1
  [phase] -> Cos3/1
  Cos3/1 -> Product3/2
  Product3/1 -> Sum4/1
  [B] -> Product4/1
  Product4/1 -> Sum4/2
  [phase] -> Sum3/1
  Constant2/1 -> Sum3/2
  Sum3/1 -> Cos4/1
  Cos4/1 -> Product4/2
  Sum5/1 -> Cos5/1
  Constant3/1 -> Sum5/2
  Cos5/1 -> Product5/2
  [phase] -> Sum5/1
  [C] -> Product5/1
  Product5/1 -> Sum4/3
  Sum4/1 -> Gain1/1
  Product2/1 -> Sum1/3
  [C] -> Product2/1
  [phase] -> Sum2/1
  Cos2/1 -> Product2/2
  Constant1/1 -> Sum2/2
  Sum2/1 -> Cos2/1
  Cos1/1 -> Product1/2
  Sum/1 -> Cos1/1
  Constant/1 -> Sum/2
  [phase] -> Sum/1
  Product1/1 -> Sum1/2
  [B] -> Product1/1
  Product/1 -> Sum1/1
  Cos/1 -> Product/2
  [phase] -> Cos/1
  [A] -> Product/1
  Phase/1 -> [phase]
  Demux/3 -> [C]
  Demux/2 -> [B]
  Demux/1 -> [A]
  ABC/1 -> Demux/1
  Mux/1 -> Delay/1
  Delay/1 -> DQ/1

== system Basic_cosimulation_circuit_simulator1/SM_Master/VSC_ITM_Intantaneous_values/Control/Power Control ==
  PQ_ref : Inport
  Vd : Inport  Port=2
  Dblk : Inport  Port=3
  Constant : Constant  Value=Vnom_peak
  Demux2 : Demux  Outputs=2
  Divide : Product  Inputs=*/
  Divide1 : Product  Inputs=*/
  Gain : Gain  Gain=3
  Gain1 : Gain  Gain=2
  Gain2 : Gain  Gain=3
  Gain3 : Gain  Gain=-2
  Mux : Mux  Inputs=2
  Scope : Scope
  Switch : Switch  Criteria=u2 > Threshold
  Transfer Fcn : TransferFcn  Commented=on  Denominator=[0.01 1]
  Out1 : Outport
  wires:
  Gain/1 -> Divide/2
  Demux2/2 -> Gain3/1
  Gain2/1 -> Divide1/2
  Gain3/1 -> Divide1/1
  Demux2/1 -> Gain1/1
  Dblk/1 -> Switch/2
  Gain1/1 -> Divide/1
  Divide/1 -> Mux/1
  Constant/1 -> Switch/3
  [Vd_power] -> Gain/1
  Divide1/1 -> Mux/2
  Mux/1 -> Out1/1
  PQ_ref/1 -> Demux2/1
  Vd/1 -> Switch/1
  Switch/1 -> Scope/1, Gain2/1, [Vd_power]

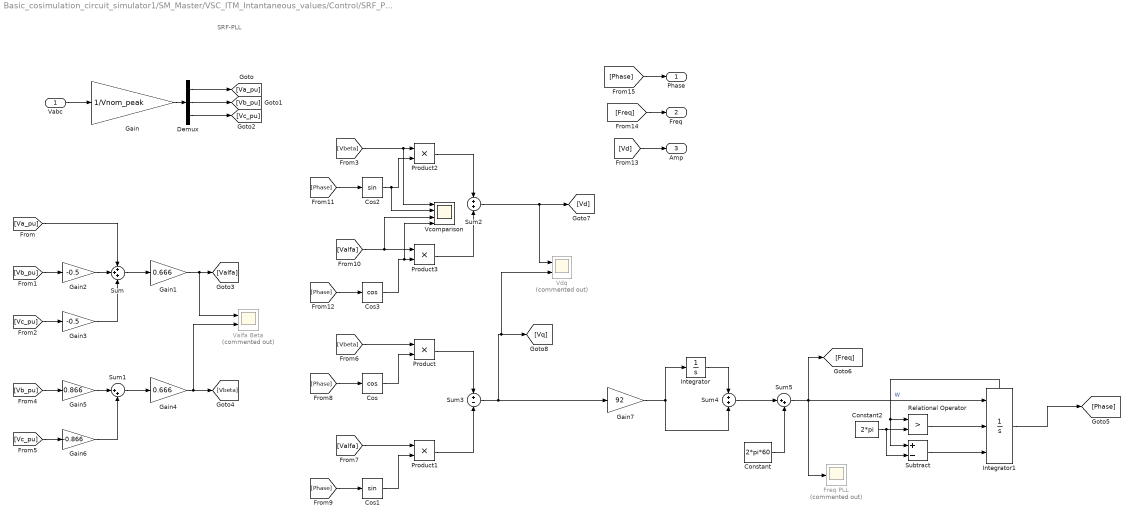
== system Basic_cosimulation_circuit_simulator1/SM_Master/VSC_ITM_Intantaneous_values/Control/SRF_PLL ==
  note: SRF-PLL
  Vabc : Inport
  Constant : Constant  Value=2*pi*60
  Constant2 : Constant  Value=2*pi
  Cos : Trigonometry  Operator=cos
  Cos1 : Trigonometry
  Cos2 : Trigonometry
  Cos3 : Trigonometry  Operator=cos
  Demux : Demux  Outputs=3
  Freq PLL : Scope  Commented=on
  Gain : Gain  Gain=1/Vnom_peak
  Gain1 : Gain  Gain=0.666
  Gain2 : Gain  Gain=-0.5
  Gain3 : Gain  Gain=-0.5
  Gain4 : Gain  Gain=0.666
  Gain5 : Gain  Gain=0.866
  Gain6 : Gain  Gain=-0.866
  Gain7 : Gain  Gain=92
  Integrator : Integrator
  Integrator1 : Integrator  ExternalReset=rising  InitialConditionSource=external  InitialCondition=sps.Phase_Init*pi/180  LimitOutput=on  ShowStatePort=on
  Product{,1..3} (4 alike) : Product
  Relational Operator : RelationalOperator  Operator=>  OutDataTypeStr=boolean  RndMeth=Nearest
  Subtract : Sum  Inputs=+-
  Sum : Sum  Inputs=+++
  Sum1 : Sum  Inputs=|++
  Sum2 : Sum  Inputs=+|+
  Sum3 : Sum  Inputs=+|-
  Sum4 : Sum  Inputs=+|+
  Sum5 : Sum  Inputs=|++
  Valfa Beta : Scope  Commented=on  NumInputPorts=2
  Vcomparison : Scope  NumInputPorts=4
  Vdq : Scope  Commented=on  NumInputPorts=2
  Phase : Outport
  Freq : Outport  Port=2
  Amp : Outport  Port=3
  wires:
  Vabc/1 -> Gain/1
  Demux/1 -> [Va_pu]
  Demux/2 -> [Vb_pu]
  Demux/3 -> [Vc_pu]
  Gain/1 -> Demux/1
  Sum/1 -> Gain1/1
  [Va_pu] -> Sum/1
  [Vb_pu] -> Gain2/1
  Gain2/1 -> Sum/2
  [Vc_pu] -> Gain3/1
  Gain3/1 -> Sum/3
  [Vc_pu] -> Gain6/1
  [Vb_pu] -> Gain5/1
  Sum1/1 -> Gain4/1
  Gain4/1 -> Valfa Beta/2, [Vbeta]
  Gain5/1 -> Sum1/1
  Gain6/1 -> Sum1/2
  [Vbeta] -> Product/1
  Product/1 -> Sum3/1
  [Valfa] -> Product1/1
  Product1/1 -> Sum3/2
  Sum3/1 -> Gain7/1, Vdq/2, [Vq]
  Gain7/1 -> Sum4/2, Integrator/1
  Integrator/1 -> Sum4/1
  Sum4/1 -> Sum5/1
  Constant/1 -> Sum5/2
  [Phase] -> Cos/1
  Cos/1 -> Product/2
  [Phase] -> Cos1/1
  Cos1/1 -> Product1/2
  Cos3/1 -> Vcomparison/4, Product3/2
  [Phase] -> Cos3/1
  Cos2/1 -> Vcomparison/2, Product2/2
  [Phase] -> Cos2/1
  Product3/1 -> Sum2/2
  [Valfa] -> Vcomparison/3, Product3/1
  Product2/1 -> Sum2/1
  [Vbeta] -> Vcomparison/1, Product2/1
  [Vd] -> Amp/1
  [Freq] -> Freq/1
  [Phase] -> Phase/1
  Gain1/1 -> Valfa Beta/1, [Valfa]
  Sum2/1 -> Vdq/1, [Vd]
  Constant2/1 -> Relational Operator/2, Subtract/2
  Integrator1/State -> Relational Operator/1, Subtract/1
  Sum5/1 -> Integrator1/1, Freq PLL/1, [Freq]  "W"
  Relational Operator/1 -> Integrator1/2
  Subtract/1 -> Integrator1/3
  Integrator1/1 -> [Phase]

== system Basic_cosimulation_circuit_simulator1/SM_Master/VSC_ITM_SFA/Control/Current Control ==
  note: Block Inputs
  Deblock : Inport
  Idq_ref : Inport  Port=2
  Idq : Inport  Port=3
  Vdq : Inport  Port=4
  Phase : Inport  Port=5
  Constant2 : Constant  Value=Vdc/2
  Delay : Delay  DelayLength=1
  Demux1 : Demux  Outputs=2
  Demux2 : Demux  Outputs=2
  Demux3 : Demux  Outputs=2
  Discrete-Time Integrator : DiscreteIntegrator  SampleTime=-1  ICPrevOutput=DiscIntNeverNeededParam  ICPrevScaledInput=DiscIntNeverNeededParam
  Discrete-Time Integrator1 : DiscreteIntegrator  SampleTime=-1  ICPrevOutput=DiscIntNeverNeededParam  ICPrevScaledInput=DiscIntNeverNeededParam
  Divide : Product  Inputs=*/
  Divide1 : Product  Inputs=*/
  Gain1 : Gain  Gain=kp_current
  Gain2 : Gain  Gain=ki_current
  Gain3 : Gain  Gain=kp_current
  Gain4 : Gain  Gain=ki_current
  Gain5 : Gain  Gain=decouple
  Gain6 : Gain  Gain=decouple
  Inverse_Park_Transformation : Subsystem
  Mux : Mux  Inputs=2
  Product : Product
  Product1 : Product
  Saturation : Saturate  UpperLimit=1.2*Inom_peak  LowerLimit=-1.2*Inom_peak
  Saturation1 : Saturate  UpperLimit=1.2*Inom_peak  LowerLimit=-1.2*Inom_peak
  Scope : Scope  Commented=on
  Subtract : Sum  Inputs=+-
  Subtract1 : Sum  Inputs=+-
  Sum1 : Sum
  Sum2 : Sum
  Sum3 : Sum  Inputs=++-
  Sum4 : Sum  Inputs=+++
  modulation : Outport
  wires:
  Sum4/1 -> Divide1/1
  Sum3/1 -> Divide/1
  Sum2/1 -> Sum4/2
  Subtract/1 -> Product/1
  Gain2/1 -> Discrete-Time Integrator/1
  [Iq] -> Gain5/1
  Gain1/1 -> Sum1/1
  [Id] -> Gain6/1
  Subtract1/1 -> Product1/2
  Gain6/1 -> Sum4/1
  Product/1 -> Gain2/1, Gain1/1
  [Vd] -> Sum3/1
  Constant2/1 -> Divide1/2, Divide/2
  Idq_ref/1 -> Demux3/1
  Mux/1 -> Delay/1
  Gain5/1 -> Sum3/3
  Sum1/1 -> Sum3/2
  Discrete-Time Integrator/1 -> Sum1/2
  Gain3/1 -> Sum2/1
  Gain4/1 -> Discrete-Time Integrator1/1
  Discrete-Time Integrator1/1 -> Sum2/2
  [Vq] -> Sum4/3
  Product1/1 -> Gain3/1, Gain4/1
  [Id] -> Subtract/2
  Divide/1 -> Mux/1
  Divide1/1 -> Mux/2
  [Iq] -> Subtract1/2
  Inverse_Park_Transformation/1(ABC) -> modulation/1
  Idq/1 -> Demux1/1
  Demux1/1 -> [Id]
  Demux1/2 -> [Iq]
  Demux2/1 -> [Vd]
  Demux2/2 -> [Vq]
  Vdq/1 -> Demux2/1
  [dblk] -> Product1/1, Product/2
  Deblock/1 -> [dblk]
  Phase/1 -> [phase_pll]
  [phase_pll] -> Inverse_Park_Transformation/2(Phase)
  Demux3/1 -> [Id_ref]
  Demux3/2 -> [Iq_ref]
  [Iq_ref] -> Saturation1/1
  [Id_ref] -> Saturation/1
  Saturation/1 -> Subtract/1
  Saturation1/1 -> Subtract1/1
  Delay/1 -> Scope/1, Inverse_Park_Transformation/1(DQ)

== system Basic_cosimulation_circuit_simulator1/SM_Master/VSC_ITM_SFA/Control/Meas_3_Wire ==
  AB : Inport
  BC : Inport  Port=2
  Gain10 : Gain  Gain=2
  Gain6 : Gain  Gain=2
  Gain7 : Gain  Gain=1/3
  Gain8 : Gain  Gain=1/3
  Gain9 : Gain  Gain=1/3
  Mux : Mux  Inputs=3
  Sum4 : Sum  Inputs=|++
  Sum5 : Sum  Inputs=-+|
  Sum6 : Sum  Inputs=--|
  ABC : Outport
  wires:
  BC/1 -> Sum4/2, Sum5/2, Gain10/1
  AB/1 -> Gain6/1, Sum5/1, Sum6/2
  Gain7/1 -> Mux/1
  Gain9/1 -> Mux/3
  Sum6/1 -> Gain9/1
  Gain6/1 -> Sum4/1
  Gain8/1 -> Mux/2
  Sum5/1 -> Gain8/1
  Gain10/1 -> Sum6/1
  Sum4/1 -> Gain7/1
  Mux/1 -> ABC/1

== system Basic_cosimulation_circuit_simulator1/SM_Master/VSC_ITM_SFA/Control/Park_Transformation ==
  note: Park Transformation
  ABC : Inport
  Phase : Inport  Port=2
  Constant{,1..3} (4 alike) : Constant  Value=2*pi/3
  Cos : Trigonometry  Operator=cos
  Cos1 : Trigonometry  Operator=cos
  Cos2 : Trigonometry  Operator=cos
  Cos3 : Trigonometry
  Cos4 : Trigonometry
  Cos5 : Trigonometry
  Delay : Delay  DelayLength=1
  Demux : Demux  Outputs=3
  Gain : Gain  Gain=0.666
  Gain1 : Gain  Gain=-0.666
  Mux : Mux  Inputs=2
  Product{,1..5} (6 alike) : Product
  Sum : Sum  Inputs=|+-
  Sum1 : Sum  Inputs=+++
  Sum2 : Sum  Inputs=|++
  Sum3 : Sum  Inputs=|+-
  Sum4 : Sum  Inputs=+++
  Sum5 : Sum  Inputs=|++
  DQ : Outport
  wires:
  ABC/1 -> Demux/1
  Demux/1 -> [A]
  Demux/2 -> [B]
  Demux/3 -> [C]
  Phase/1 -> [phase]
  [A] -> Product/1
  [phase] -> Cos/1
  Cos/1 -> Product/2
  Product/1 -> Sum1/1
  [B] -> Product1/1
  Product1/1 -> Sum1/2
  [phase] -> Sum/1
  Constant/1 -> Sum/2
  Sum/1 -> Cos1/1
  Cos1/1 -> Product1/2
  Sum2/1 -> Cos2/1
  Constant1/1 -> Sum2/2
  Cos2/1 -> Product2/2
  [phase] -> Sum2/1
  [C] -> Product2/1
  Product2/1 -> Sum1/3
  Sum4/1 -> Gain1/1
  Product5/1 -> Sum4/3
  [C] -> Product5/1
  [phase] -> Sum5/1
  Cos5/1 -> Product5/2
  Constant3/1 -> Sum5/2
  Sum5/1 -> Cos5/1
  Cos4/1 -> Product4/2
  Sum3/1 -> Cos4/1
  Constant2/1 -> Sum3/2
  [phase] -> Sum3/1
  Product4/1 -> Sum4/2
  [B] -> Product4/1
  Product3/1 -> Sum4/1
  Cos3/1 -> Product3/2
  [phase] -> Cos3/1
  [A] -> Product3/1
  Sum1/1 -> Gain/1
  Gain/1 -> [D]
  Gain1/1 -> [Q]
  [D] -> Mux/1
  [Q] -> Mux/2
  Mux/1 -> Delay/1
  Delay/1 -> DQ/1

== system Basic_cosimulation_circuit_simulator1/SM_Master/VSC_ITM_SFA/Control/Park_Transformation1 ==
  note: Park Transformation
  ABC : Inport
  Phase : Inport  Port=2
  Constant{,1..3} (4 alike) : Constant  Value=2*pi/3
  Cos : Trigonometry  Operator=cos
  Cos1 : Trigonometry  Operator=cos
  Cos2 : Trigonometry  Operator=cos
  Cos3 : Trigonometry
  Cos4 : Trigonometry
  Cos5 : Trigonometry
  Delay : Delay  DelayLength=1
  Demux : Demux  Outputs=3
  Gain : Gain  Gain=0.666
  Gain1 : Gain  Gain=-0.666
  Mux : Mux  Inputs=2
  Product{,1..5} (6 alike) : Product
  Sum : Sum  Inputs=|+-
  Sum1 : Sum  Inputs=+++
  Sum2 : Sum  Inputs=|++
  Sum3 : Sum  Inputs=|+-
  Sum4 : Sum  Inputs=+++
  Sum5 : Sum  Inputs=|++
  DQ : Outport
  wires:
  [Q] -> Mux/2
  [D] -> Mux/1
  Gain1/1 -> [Q]
  Gain/1 -> [D]
  Sum1/1 -> Gain/1
  [A] -> Product3/1
  [phase] -> Cos3/1
  Cos3/1 -> Product3/2
  Product3/1 -> Sum4/1
  [B] -> Product4/1
  Product4/1 -> Sum4/2
  [phase] -> Sum3/1
  Constant2/1 -> Sum3/2
  Sum3/1 -> Cos4/1
  Cos4/1 -> Product4/2
  Sum5/1 -> Cos5/1
  Constant3/1 -> Sum5/2
  Cos5/1 -> Product5/2
  [phase] -> Sum5/1
  [C] -> Product5/1
  Product5/1 -> Sum4/3
  Sum4/1 -> Gain1/1
  Product2/1 -> Sum1/3
  [C] -> Product2/1
  [phase] -> Sum2/1
  Cos2/1 -> Product2/2
  Constant1/1 -> Sum2/2
  Sum2/1 -> Cos2/1
  Cos1/1 -> Product1/2
  Sum/1 -> Cos1/1
  Constant/1 -> Sum/2
  [phase] -> Sum/1
  Product1/1 -> Sum1/2
  [B] -> Product1/1
  Product/1 -> Sum1/1
  Cos/1 -> Product/2
  [phase] -> Cos/1
  [A] -> Product/1
  Phase/1 -> [phase]
  Demux/3 -> [C]
  Demux/2 -> [B]
  Demux/1 -> [A]
  ABC/1 -> Demux/1
  Mux/1 -> Delay/1
  Delay/1 -> DQ/1

== system Basic_cosimulation_circuit_simulator1/SM_Master/VSC_ITM_SFA/Control/Power Control ==
  PQ_ref : Inport
  Vd : Inport  Port=2
  Dblk : Inport  Port=3
  Constant : Constant  Value=Vnom_peak
  Constant1 : Constant  Value=eps
  Demux2 : Demux  Outputs=2
  Divide : Product  Inputs=*/
  Divide1 : Product  Inputs=*/
  Gain : Gain  Gain=3
  Gain1 : Gain  Gain=2
  Gain2 : Gain  Gain=3
  Gain3 : Gain  Gain=-2
  Mux : Mux  Inputs=2
  Saturation : Saturate  UpperLimit=10e3  LowerLimit=-10e3
  Scope : Scope
  Switch : Switch  Criteria=u2 > Threshold
  Switch1 : Switch  Criteria=u2 ~= 0
  Transfer Fcn : TransferFcn  Commented=on  Denominator=[0.01 1]
  Out1 : Outport
  wires:
  Gain/1 -> Divide/2
  Demux2/2 -> Gain3/1
  Gain2/1 -> Divide1/2
  Gain3/1 -> Divide1/1
  Demux2/1 -> Gain1/1
  Dblk/1 -> Switch/2
  Gain1/1 -> Divide/1
  Divide/1 -> Mux/1
  Constant/1 -> Switch/3
  [Vd_power] -> Gain/1
  Divide1/1 -> Mux/2
  Mux/1 -> Saturation/1
  PQ_ref/1 -> Demux2/1
  Switch/1 -> Scope/1, Gain2/1, [Vd_power]
  Constant1/1 -> Switch1/3
  Vd/1 -> Switch1/1, Switch1/2
  Switch1/1 -> Switch/1
  Saturation/1 -> Out1/1

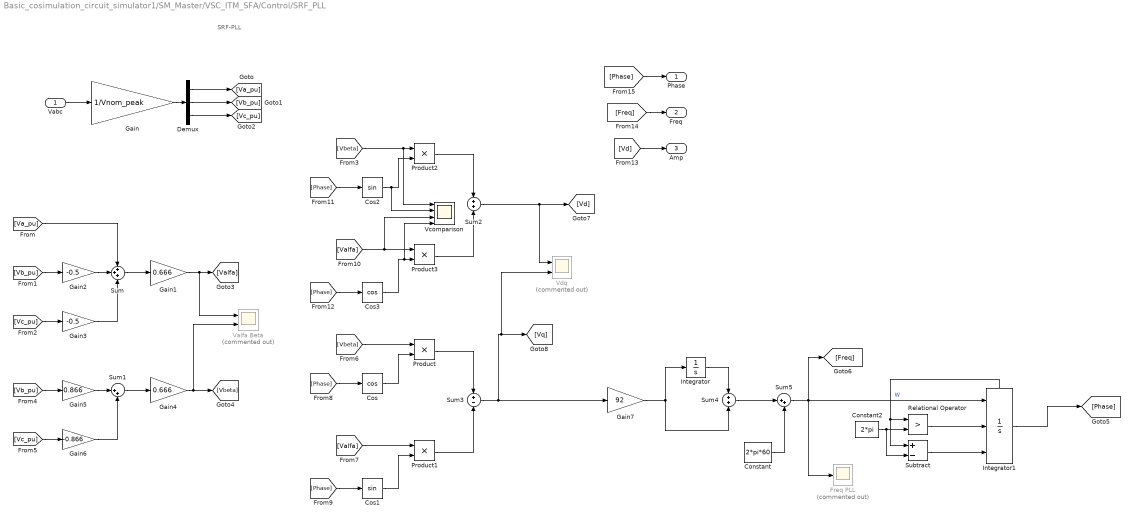
== system Basic_cosimulation_circuit_simulator1/SM_Master/VSC_ITM_SFA/Control/SRF_PLL ==
  note: SRF-PLL
  Vabc : Inport
  Constant : Constant  Value=2*pi*60
  Constant2 : Constant  Value=2*pi
  Cos : Trigonometry  Operator=cos
  Cos1 : Trigonometry
  Cos2 : Trigonometry
  Cos3 : Trigonometry  Operator=cos
  Demux : Demux  Outputs=3
  Freq PLL : Scope  Commented=on
  Gain : Gain  Gain=1/Vnom_peak
  Gain1 : Gain  Gain=0.666
  Gain2 : Gain  Gain=-0.5
  Gain3 : Gain  Gain=-0.5
  Gain4 : Gain  Gain=0.666
  Gain5 : Gain  Gain=0.866
  Gain6 : Gain  Gain=-0.866
  Gain7 : Gain  Gain=92
  Integrator : Integrator
  Integrator1 : Integrator  ExternalReset=rising  InitialConditionSource=external  InitialCondition=sps.Phase_Init*pi/180  LimitOutput=on  ShowStatePort=on
  Product{,1..3} (4 alike) : Product
  Relational Operator : RelationalOperator  Operator=>  OutDataTypeStr=boolean  RndMeth=Nearest
  Subtract : Sum  Inputs=+-
  Sum : Sum  Inputs=+++
  Sum1 : Sum  Inputs=|++
  Sum2 : Sum  Inputs=+|+
  Sum3 : Sum  Inputs=+|-
  Sum4 : Sum  Inputs=+|+
  Sum5 : Sum  Inputs=|++
  Valfa Beta : Scope  Commented=on  NumInputPorts=2
  Vcomparison : Scope  NumInputPorts=4
  Vdq : Scope  Commented=on  NumInputPorts=2
  Phase : Outport
  Freq : Outport  Port=2
  Amp : Outport  Port=3
  wires:
  Vabc/1 -> Gain/1
  Demux/1 -> [Va_pu]
  Demux/2 -> [Vb_pu]
  Demux/3 -> [Vc_pu]
  Gain/1 -> Demux/1
  Sum/1 -> Gain1/1
  [Va_pu] -> Sum/1
  [Vb_pu] -> Gain2/1
  Gain2/1 -> Sum/2
  [Vc_pu] -> Gain3/1
  Gain3/1 -> Sum/3
  [Vc_pu] -> Gain6/1
  [Vb_pu] -> Gain5/1
  Sum1/1 -> Gain4/1
  Gain4/1 -> Valfa Beta/2, [Vbeta]
  Gain5/1 -> Sum1/1
  Gain6/1 -> Sum1/2
  [Vbeta] -> Product/1
  Product/1 -> Sum3/1
  [Valfa] -> Product1/1
  Product1/1 -> Sum3/2
  Sum3/1 -> Gain7/1, Vdq/2, [Vq]
  Gain7/1 -> Sum4/2, Integrator/1
  Integrator/1 -> Sum4/1
  Sum4/1 -> Sum5/1
  Constant/1 -> Sum5/2
  [Phase] -> Cos/1
  Cos/1 -> Product/2
  [Phase] -> Cos1/1
  Cos1/1 -> Product1/2
  Cos3/1 -> Vcomparison/4, Product3/2
  [Phase] -> Cos3/1
  Cos2/1 -> Vcomparison/2, Product2/2
  [Phase] -> Cos2/1
  Product3/1 -> Sum2/2
  [Valfa] -> Vcomparison/3, Product3/1
  Product2/1 -> Sum2/1
  [Vbeta] -> Vcomparison/1, Product2/1
  [Vd] -> Amp/1
  [Freq] -> Freq/1
  [Phase] -> Phase/1
  Gain1/1 -> Valfa Beta/1, [Valfa]
  Sum2/1 -> Vdq/1, [Vd]
  Constant2/1 -> Relational Operator/2, Subtract/2
  Integrator1/State -> Relational Operator/1, Subtract/1
  Sum5/1 -> Integrator1/1, Freq PLL/1, [Freq]  "W"
  Relational Operator/1 -> Integrator1/2
  Subtract/1 -> Integrator1/3
  Integrator1/1 -> [Phase]
